simulink model "MLP_Final_Golden"  (R2015b)
settings: Solver=FixedStepDiscrete  SolverMode=SingleTasking  StartTime=0.0  StopTime=1e-2  RelTol=1e-3
undefined symbols (not defined in the file): input_sample_time, system_sample_time
libraries: shlslibv1 x1948
(part 5 of 11)

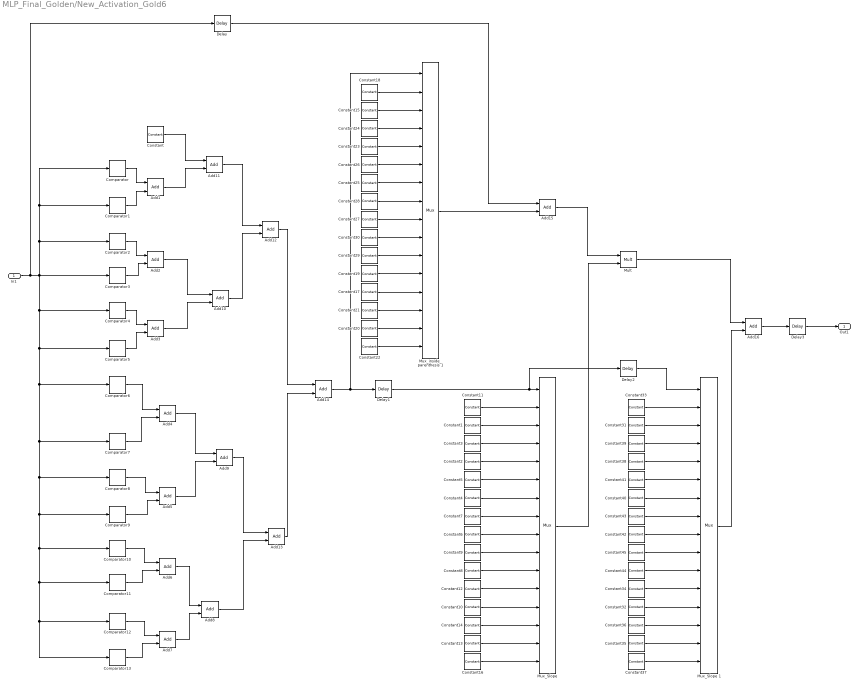
== system MLP_Final_Golden/New_Activation_Gold6 ==
  In1 : Inport
  Add{1..14} (14 alike) : shlslibv1/Math Functions/Add  syn_add_opr=++  syn_out_f=Specify  syn_out_wl=5  syn_out_fl=0  syn_out_dt=unsigned  syn_out_sat=off  syn_out_rnd=Nearest  synBlockType=primitive  synLatency=0  synBlockId=96  syn_sum_of_rows=off  syn_inh_port=off  syn_inh_st=on  syn_inh_stf=1  syn_en_pipe=on  syn_pipe_stg=3  syn_flow_ctrl=off
  Add15 : shlslibv1/Math Functions/Add  syn_add_opr=+-  syn_out_f=Specify  syn_out_wl=32  syn_out_fl=16  syn_out_dt=signed  syn_out_sat=off  syn_out_rnd=Floor (Truncate)  synBlockType=primitive  synLatency=0  synBlockId=96  syn_sum_of_rows=off  syn_inh_port=off  syn_inh_st=on  syn_inh_stf=1  syn_en_pipe=on  syn_pipe_stg=3  syn_flow_ctrl=off
  Add16 : shlslibv1/Math Functions/Add  syn_add_opr=++  syn_out_f=Specify  syn_out_wl=32  syn_out_fl=16  syn_out_dt=signed  syn_out_sat=off  syn_out_rnd=Floor (Truncate)  synBlockType=primitive  synLatency=0  synBlockId=96  syn_sum_of_rows=off  syn_inh_port=off  syn_inh_st=on  syn_inh_stf=1  syn_en_pipe=on  syn_pipe_stg=3  syn_flow_ctrl=off
  Comparator : shlslibv1/Math Functions/Comparator  syn_comp_opr=a>=b  syn_comp_const=on  syn_comp_val=6.5  syn_en_se=off  synBlockType=primitive  synLatency=0  synBlockId=14
  Comparator1 : shlslibv1/Math Functions/Comparator  syn_comp_opr=a>=b  syn_comp_const=on  syn_comp_val=5.5  syn_en_se=off  synBlockType=primitive  synLatency=0  synBlockId=14
  Comparator10 : shlslibv1/Math Functions/Comparator  syn_comp_opr=a>=b  syn_comp_const=on  syn_comp_val=-3.5  syn_en_se=off  synBlockType=primitive  synLatency=0  synBlockId=14
  Comparator11 : shlslibv1/Math Functions/Comparator  syn_comp_opr=a>=b  syn_comp_const=on  syn_comp_val=-4.5  syn_en_se=off  synBlockType=primitive  synLatency=0  synBlockId=14
  Comparator12 : shlslibv1/Math Functions/Comparator  syn_comp_opr=a>=b  syn_comp_const=on  syn_comp_val=-5.5  syn_en_se=off  synBlockType=primitive  synLatency=0  synBlockId=14
  Comparator13 : shlslibv1/Math Functions/Comparator  syn_comp_opr=a>=b  syn_comp_const=on  syn_comp_val=-6.5  syn_en_se=off  synBlockType=primitive  synLatency=0  synBlockId=14
  Comparator2 : shlslibv1/Math Functions/Comparator  syn_comp_opr=a>=b  syn_comp_const=on  syn_comp_val=4.5  syn_en_se=off  synBlockType=primitive  synLatency=0  synBlockId=14
  Comparator3 : shlslibv1/Math Functions/Comparator  syn_comp_opr=a>=b  syn_comp_const=on  syn_comp_val=3.5  syn_en_se=off  synBlockType=primitive  synLatency=0  synBlockId=14
  Comparator4 : shlslibv1/Math Functions/Comparator  syn_comp_opr=a>=b  syn_comp_const=on  syn_comp_val=2.5  syn_en_se=off  synBlockType=primitive  synLatency=0  synBlockId=14
  Comparator5 : shlslibv1/Math Functions/Comparator  syn_comp_opr=a>=b  syn_comp_const=on  syn_comp_val=1.5  syn_en_se=off  synBlockType=primitive  synLatency=0  synBlockId=14
  Comparator6 : shlslibv1/Math Functions/Comparator  syn_comp_opr=a>=b  syn_comp_const=on  syn_comp_val=0.5  syn_en_se=off  synBlockType=primitive  synLatency=0  synBlockId=14
  Comparator7 : shlslibv1/Math Functions/Comparator  syn_comp_opr=a>=b  syn_comp_const=on  syn_comp_val=-0.5  syn_en_se=off  synBlockType=primitive  synLatency=0  synBlockId=14
  Comparator8 : shlslibv1/Math Functions/Comparator  syn_comp_opr=a>=b  syn_comp_const=on  syn_comp_val=-1.5  syn_en_se=off  synBlockType=primitive  synLatency=0  synBlockId=14
  Comparator9 : shlslibv1/Math Functions/Comparator  syn_comp_opr=a>=b  syn_comp_const=on  syn_comp_val=-2.5  syn_en_se=off  synBlockType=primitive  synLatency=0  synBlockId=14
  Constant : shlslibv1/Sources/Constant  syn_cst_val=0  syn_cst_format=Specify  syn_cst_wl=5  syn_cst_fl=0  syn_cst_dt=unsigned  syn_cst_rnd=on  syn_cst_st=-1  synBlockType=primitive  synLatency=0  synBlockId=15
  Constant1 : shlslibv1/Sources/Constant  syn_cst_val=0.0025  syn_cst_format=Specify  syn_cst_wl=32  syn_cst_fl=16  syn_cst_dt=unsigned  syn_cst_rnd=on  syn_cst_st=-1  synBlockType=primitive  synLatency=0  synBlockId=15
  Constant10 : shlslibv1/Sources/Constant  syn_cst_val=0.0177  syn_cst_format=Specify  syn_cst_wl=32  syn_cst_fl=16  syn_cst_dt=unsigned  syn_cst_rnd=on  syn_cst_st=-1  synBlockType=primitive  synLatency=0  synBlockId=15
  Constant{11,16,18,22,33} (5 alike) : shlslibv1/Sources/Constant  syn_cst_val=0  syn_cst_format=Specify  syn_cst_wl=32  syn_cst_fl=16  syn_cst_dt=unsigned  syn_cst_rnd=on  syn_cst_st=-1  synBlockType=primitive  synLatency=0  synBlockId=15
  Constant12 : shlslibv1/Sources/Constant  syn_cst_val=0.0452  syn_cst_format=Specify  syn_cst_wl=32  syn_cst_fl=16  syn_cst_dt=unsigned  syn_cst_rnd=on  syn_cst_st=-1  synBlockType=primitive  synLatency=0  synBlockId=15
  Constant13 : shlslibv1/Sources/Constant  syn_cst_val=0.0025  syn_cst_format=Specify  syn_cst_wl=32  syn_cst_fl=16  syn_cst_dt=unsigned  syn_cst_rnd=on  syn_cst_st=-1  synBlockType=primitive  synLatency=0  synBlockId=15
  Constant14 : shlslibv1/Sources/Constant  syn_cst_val=0.0066  syn_cst_format=Specify  syn_cst_wl=32  syn_cst_fl=16  syn_cst_dt=unsigned  syn_cst_rnd=on  syn_cst_st=-1  synBlockType=primitive  synLatency=0  synBlockId=15
  Constant15 : shlslibv1/Sources/Constant  syn_cst_val=-6.5  syn_cst_format=Specify  syn_cst_wl=32  syn_cst_fl=16  syn_cst_dt=unsigned  syn_cst_rnd=on  syn_cst_st=-1  synBlockType=primitive  synLatency=0  synBlockId=15
  Constant17 : shlslibv1/Sources/Constant  syn_cst_val=3.5  syn_cst_format=Specify  syn_cst_wl=32  syn_cst_fl=16  syn_cst_dt=unsigned  syn_cst_rnd=on  syn_cst_st=-1  synBlockType=primitive  synLatency=0  synBlockId=15
  Constant19 : shlslibv1/Sources/Constant  syn_cst_val=2.5  syn_cst_format=Specify  syn_cst_wl=32  syn_cst_fl=16  syn_cst_dt=unsigned  syn_cst_rnd=on  syn_cst_st=-1  synBlockType=primitive  synLatency=0  synBlockId=15
  Constant2 : shlslibv1/Sources/Constant  syn_cst_val=0.0177  syn_cst_format=Specify  syn_cst_wl=32  syn_cst_fl=16  syn_cst_dt=unsigned  syn_cst_rnd=on  syn_cst_st=-1  synBlockType=primitive  synLatency=0  synBlockId=15
  Constant20 : shlslibv1/Sources/Constant  syn_cst_val=5.5  syn_cst_format=Specify  syn_cst_wl=32  syn_cst_fl=16  syn_cst_dt=unsigned  syn_cst_rnd=on  syn_cst_st=-1  synBlockType=primitive  synLatency=0  synBlockId=15
  Constant21 : shlslibv1/Sources/Constant  syn_cst_val=4.5  syn_cst_format=Specify  syn_cst_wl=32  syn_cst_fl=16  syn_cst_dt=unsigned  syn_cst_rnd=on  syn_cst_st=-1  synBlockType=primitive  synLatency=0  synBlockId=15
  Constant23 : shlslibv1/Sources/Constant  syn_cst_val=-4.5  syn_cst_format=Specify  syn_cst_wl=32  syn_cst_fl=16  syn_cst_dt=unsigned  syn_cst_rnd=on  syn_cst_st=-1  synBlockType=primitive  synLatency=0  synBlockId=15
  Constant24 : shlslibv1/Sources/Constant  syn_cst_val=-5.5  syn_cst_format=Specify  syn_cst_wl=32  syn_cst_fl=16  syn_cst_dt=unsigned  syn_cst_rnd=on  syn_cst_st=-1  synBlockType=primitive  synLatency=0  synBlockId=15
  Constant25 : shlslibv1/Sources/Constant  syn_cst_val=-2.5  syn_cst_format=Specify  syn_cst_wl=32  syn_cst_fl=16  syn_cst_dt=unsigned  syn_cst_rnd=on  syn_cst_st=-1  synBlockType=primitive  synLatency=0  synBlockId=15
  Constant26 : shlslibv1/Sources/Constant  syn_cst_val=-3.5  syn_cst_format=Specify  syn_cst_wl=32  syn_cst_fl=16  syn_cst_dt=unsigned  syn_cst_rnd=on  syn_cst_st=-1  synBlockType=primitive  synLatency=0  synBlockId=15
  Constant27 : shlslibv1/Sources/Constant  syn_cst_val=-0.5  syn_cst_format=Specify  syn_cst_wl=32  syn_cst_fl=16  syn_cst_dt=unsigned  syn_cst_rnd=on  syn_cst_st=-1  synBlockType=primitive  synLatency=0  synBlockId=15
  Constant28 : shlslibv1/Sources/Constant  syn_cst_val=-1.5  syn_cst_format=Specify  syn_cst_wl=32  syn_cst_fl=16  syn_cst_dt=unsigned  syn_cst_rnd=on  syn_cst_st=-1  synBlockType=primitive  synLatency=0  synBlockId=15
  Constant29 : shlslibv1/Sources/Constant  syn_cst_val=1.5  syn_cst_format=Specify  syn_cst_wl=32  syn_cst_fl=16  syn_cst_dt=unsigned  syn_cst_rnd=on  syn_cst_st=-1  synBlockType=primitive  synLatency=0  synBlockId=15
  Constant3 : shlslibv1/Sources/Constant  syn_cst_val=0.0066  syn_cst_format=Specify  syn_cst_wl=32  syn_cst_fl=16  syn_cst_dt=unsigned  syn_cst_rnd=on  syn_cst_st=-1  synBlockType=primitive  synLatency=0  synBlockId=15
  Constant30 : shlslibv1/Sources/Constant  syn_cst_val=0.5  syn_cst_format=Specify  syn_cst_wl=32  syn_cst_fl=16  syn_cst_dt=unsigned  syn_cst_rnd=on  syn_cst_st=-1  synBlockType=primitive  synLatency=0  synBlockId=15
  Constant31 : shlslibv1/Sources/Constant  syn_cst_val=0.0015  syn_cst_format=Specify  syn_cst_wl=32  syn_cst_fl=16  syn_cst_dt=unsigned  syn_cst_rnd=on  syn_cst_st=-1  synBlockType=primitive  synLatency=0  synBlockId=15
  Constant32 : shlslibv1/Sources/Constant  syn_cst_val=0.9707  syn_cst_format=Specify  syn_cst_wl=32  syn_cst_fl=16  syn_cst_dt=unsigned  syn_cst_rnd=on  syn_cst_st=-1  synBlockType=primitive  synLatency=0  synBlockId=15
  Constant34 : shlslibv1/Sources/Constant  syn_cst_val=0.9241  syn_cst_format=Specify  syn_cst_wl=32  syn_cst_fl=16  syn_cst_dt=unsigned  syn_cst_rnd=on  syn_cst_st=-1  synBlockType=primitive  synLatency=0  synBlockId=15
  Constant35 : shlslibv1/Sources/Constant  syn_cst_val=0.9959  syn_cst_format=Specify  syn_cst_wl=32  syn_cst_fl=16  syn_cst_dt=unsigned  syn_cst_rnd=on  syn_cst_st=-1  synBlockType=primitive  synLatency=0  synBlockId=15
  Constant36 : shlslibv1/Sources/Constant  syn_cst_val=0.9890  syn_cst_format=Specify  syn_cst_wl=32  syn_cst_fl=16  syn_cst_dt=unsigned  syn_cst_rnd=on  syn_cst_st=-1  synBlockType=primitive  synLatency=0  synBlockId=15
  Constant37 : shlslibv1/Sources/Constant  syn_cst_val=1  syn_cst_format=Specify  syn_cst_wl=32  syn_cst_fl=16  syn_cst_dt=unsigned  syn_cst_rnd=on  syn_cst_st=-1  synBlockType=primitive  synLatency=0  synBlockId=15
  Constant38 : shlslibv1/Sources/Constant  syn_cst_val=0.011  syn_cst_format=Specify  syn_cst_wl=32  syn_cst_fl=16  syn_cst_dt=unsigned  syn_cst_rnd=on  syn_cst_st=-1  synBlockType=primitive  synLatency=0  synBlockId=15
  Constant39 : shlslibv1/Sources/Constant  syn_cst_val=0.0041  syn_cst_format=Specify  syn_cst_wl=32  syn_cst_fl=16  syn_cst_dt=unsigned  syn_cst_rnd=on  syn_cst_st=-1  synBlockType=primitive  synLatency=0  synBlockId=15
  Constant4 : shlslibv1/Sources/Constant  syn_cst_val=0.1050  syn_cst_format=Specify  syn_cst_wl=32  syn_cst_fl=16  syn_cst_dt=unsigned  syn_cst_rnd=on  syn_cst_st=-1  synBlockType=primitive  synLatency=0  synBlockId=15
  Constant40 : shlslibv1/Sources/Constant  syn_cst_val=0.0759  syn_cst_format=Specify  syn_cst_wl=32  syn_cst_fl=16  syn_cst_dt=unsigned  syn_cst_rnd=on  syn_cst_st=-1  synBlockType=primitive  synLatency=0  synBlockId=15
  Constant41 : shlslibv1/Sources/Constant  syn_cst_val=0.0293  syn_cst_format=Specify  syn_cst_wl=32  syn_cst_fl=16  syn_cst_dt=unsigned  syn_cst_rnd=on  syn_cst_st=-1  synBlockType=primitive  synLatency=0  synBlockId=15
  Constant42 : shlslibv1/Sources/Constant  syn_cst_val=0.3775  syn_cst_format=Specify  syn_cst_wl=32  syn_cst_fl=16  syn_cst_dt=unsigned  syn_cst_rnd=on  syn_cst_st=-1  synBlockType=primitive  synLatency=0  synBlockId=15
  Constant43 : shlslibv1/Sources/Constant  syn_cst_val=0.1824  syn_cst_format=Specify  syn_cst_wl=32  syn_cst_fl=16  syn_cst_dt=unsigned  syn_cst_rnd=on  syn_cst_st=-1  synBlockType=primitive  synLatency=0  synBlockId=15
  Constant44 : shlslibv1/Sources/Constant  syn_cst_val=0.8176  syn_cst_format=Specify  syn_cst_wl=32  syn_cst_fl=16  syn_cst_dt=unsigned  syn_cst_rnd=on  syn_cst_st=-1  synBlockType=primitive  synLatency=0  synBlockId=15
  Constant45 : shlslibv1/Sources/Constant  syn_cst_val=0.6225  syn_cst_format=Specify  syn_cst_wl=32  syn_cst_fl=16  syn_cst_dt=unsigned  syn_cst_rnd=on  syn_cst_st=-1  synBlockType=primitive  synLatency=0  synBlockId=15
  Constant5 : shlslibv1/Sources/Constant  syn_cst_val=0.0452  syn_cst_format=Specify  syn_cst_wl=32  syn_cst_fl=16  syn_cst_dt=unsigned  syn_cst_rnd=on  syn_cst_st=-1  synBlockType=primitive  synLatency=0  synBlockId=15
  Constant6 : shlslibv1/Sources/Constant  syn_cst_val=0.25  syn_cst_format=Specify  syn_cst_wl=32  syn_cst_fl=16  syn_cst_dt=unsigned  syn_cst_rnd=on  syn_cst_st=-1  synBlockType=primitive  synLatency=0  synBlockId=15
  Constant7 : shlslibv1/Sources/Constant  syn_cst_val=0.1966  syn_cst_format=Specify  syn_cst_wl=32  syn_cst_fl=16  syn_cst_dt=unsigned  syn_cst_rnd=on  syn_cst_st=-1  synBlockType=primitive  synLatency=0  synBlockId=15
  Constant8 : shlslibv1/Sources/Constant  syn_cst_val=0.1050  syn_cst_format=Specify  syn_cst_wl=32  syn_cst_fl=16  syn_cst_dt=unsigned  syn_cst_rnd=on  syn_cst_st=-1  synBlockType=primitive  synLatency=0  synBlockId=15
  Constant9 : shlslibv1/Sources/Constant  syn_cst_val=0.1966  syn_cst_format=Specify  syn_cst_wl=32  syn_cst_fl=16  syn_cst_dt=unsigned  syn_cst_rnd=on  syn_cst_st=-1  synBlockType=primitive  synLatency=0  synBlockId=15
  Delay : shlslibv1/Memories/Delay  syn_delay_val=12  synBlockType=primitive  synLatency=12  synBlockId=104
  Delay1 : shlslibv1/Memories/Delay  syn_delay_val=3  synBlockType=primitive  synLatency=3  synBlockId=104
  Delay2 : shlslibv1/Memories/Delay  syn_delay_val=6  synBlockType=primitive  synLatency=6  synBlockId=104
  Delay3 : shlslibv1/Memories/Delay  syn_delay_val=5  synBlockType=primitive  synLatency=5  synBlockId=104
  Mult : shlslibv1/Math Functions/Mult  syn_out_f=Specify  syn_out_wl=32  syn_out_fl=16  syn_out_dt=signed  syn_out_sat=off  syn_out_rnd=Floor (Truncate)  syn_inh_port=off  syn_inh_st=off  syn_inh_stf=1  syn_en_pipe=on  syn_pipe_stg=6  syn_flow_ctrl=off  synBlockType=primitive  synLatency=0  synBlockId=3  syn_opr_mode=1
  "Mux_Slope " : shlslibv1/Signal Operations/Mux  syn_in_nb=15  syn_out_f=Specify  syn_out_wl=32  syn_out_fl=16  syn_out_dt=signed  syn_en_se=off  synBlockType=primitive  synLatency=0  synBlockId=16
  Mux_Slope 1 : shlslibv1/Signal Operations/Mux  syn_in_nb=15  syn_out_f=Specify  syn_out_wl=32  syn_out_fl=16  syn_out_dt=signed  syn_en_se=off  synBlockType=primitive  synLatency=0  synBlockId=16
  Mux_inside_parenthesis 1 : shlslibv1/Signal Operations/Mux  syn_in_nb=15  syn_out_f=Specify  syn_out_wl=32  syn_out_fl=16  syn_out_dt=signed  syn_en_se=off  synBlockType=primitive  synLatency=0  synBlockId=16
  Out1 : Outport
  wires:
  Add12/1 -> Add14/1
  Constant14/1 -> "Mux_Slope "/14
  Constant13/1 -> "Mux_Slope "/15
  Comparator/1 -> Add1/1
  Add4/1 -> Add9/1
  Delay/1 -> Add15/1
  Constant5/1 -> "Mux_Slope "/6
  Comparator13/1 -> Add7/2
  Constant/1 -> Add11/1
  Constant29/1 -> Mux_inside_parenthesis 1/11
  Add2/1 -> Add10/1
  Add13/1 -> Add14/2
  Constant20/1 -> Mux_inside_parenthesis 1/15
  Constant23/1 -> Mux_inside_parenthesis 1/5
  Constant17/1 -> Mux_inside_parenthesis 1/13
  Add6/1 -> Add8/1
  Comparator9/1 -> Add5/2
  Constant3/1 -> "Mux_Slope "/4
  Constant2/1 -> "Mux_Slope "/5
  In1/1 -> Delay/1, Comparator7/1, Comparator8/1, Comparator12/1, Comparator13/1, Comparator11/1, Comparator10/1, Comparator9/1, Comparator6/1, Comparator5/1, Comparator4/1, Comparator3/1, Comparator2/1, Comparator1/1, Comparator/1
  Comparator2/1 -> Add2/1
  Comparator11/1 -> Add6/2
  Add11/1 -> Add12/1
  Comparator1/1 -> Add1/2
  Constant22/1 -> Mux_inside_parenthesis 1/16
  Add3/1 -> Add10/2
  Add10/1 -> Add12/2
  Comparator12/1 -> Add7/1
  Comparator8/1 -> Add5/1
  Constant9/1 -> "Mux_Slope "/10
  Add7/1 -> Add8/2
  Add14/1 -> Delay1/1, Mux_inside_parenthesis 1/1
  Constant42/1 -> Mux_Slope 1/9
  Constant1/1 -> "Mux_Slope "/3
  Constant16/1 -> "Mux_Slope "/16
  Constant24/1 -> Mux_inside_parenthesis 1/4
  Constant19/1 -> Mux_inside_parenthesis 1/12
  Constant39/1 -> Mux_Slope 1/4
  Constant41/1 -> Mux_Slope 1/6
  Constant38/1 -> Mux_Slope 1/5
  Delay1/1 -> Delay2/1, "Mux_Slope "/1
  Constant30/1 -> Mux_inside_parenthesis 1/10
  Constant45/1 -> Mux_Slope 1/10
  Constant44/1 -> Mux_Slope 1/11
  Constant34/1 -> Mux_Slope 1/12
  Constant28/1 -> Mux_inside_parenthesis 1/8
  Constant26/1 -> Mux_inside_parenthesis 1/6
  Constant21/1 -> Mux_inside_parenthesis 1/14
  Constant8/1 -> "Mux_Slope "/11
  Constant12/1 -> "Mux_Slope "/12
  Constant10/1 -> "Mux_Slope "/13
  Comparator5/1 -> Add3/2
  Constant27/1 -> Mux_inside_parenthesis 1/9
  Constant18/1 -> Mux_inside_parenthesis 1/2
  Comparator4/1 -> Add3/1
  Comparator10/1 -> Add6/1
  Constant11/1 -> "Mux_Slope "/2
  "Mux_Slope "/1 -> Mult/2
  Constant15/1 -> Mux_inside_parenthesis 1/3
  Constant32/1 -> Mux_Slope 1/13
  Constant36/1 -> Mux_Slope 1/14
  Constant35/1 -> Mux_Slope 1/15
  Constant31/1 -> Mux_Slope 1/3
  Constant25/1 -> Mux_inside_parenthesis 1/7
  Constant37/1 -> Mux_Slope 1/16
  Constant33/1 -> Mux_Slope 1/2
  Constant43/1 -> Mux_Slope 1/8
  Constant40/1 -> Mux_Slope 1/7
  Delay2/1 -> Mux_Slope 1/1
  Mult/1 -> Add16/1
  Add1/1 -> Add11/2
  Add9/1 -> Add13/1
  Constant6/1 -> "Mux_Slope "/9
  Constant4/1 -> "Mux_Slope "/7
  Add5/1 -> Add9/2
  Comparator6/1 -> Add4/1
  Comparator7/1 -> Add4/2
  Comparator3/1 -> Add2/2
  Mux_Slope 1/1 -> Add16/2
  Add8/1 -> Add13/2
  Mux_inside_parenthesis 1/1 -> Add15/2
  Constant7/1 -> "Mux_Slope "/8
  Add15/1 -> Mult/1
  Delay3/1 -> Out1/1
  Add16/1 -> Delay3/1

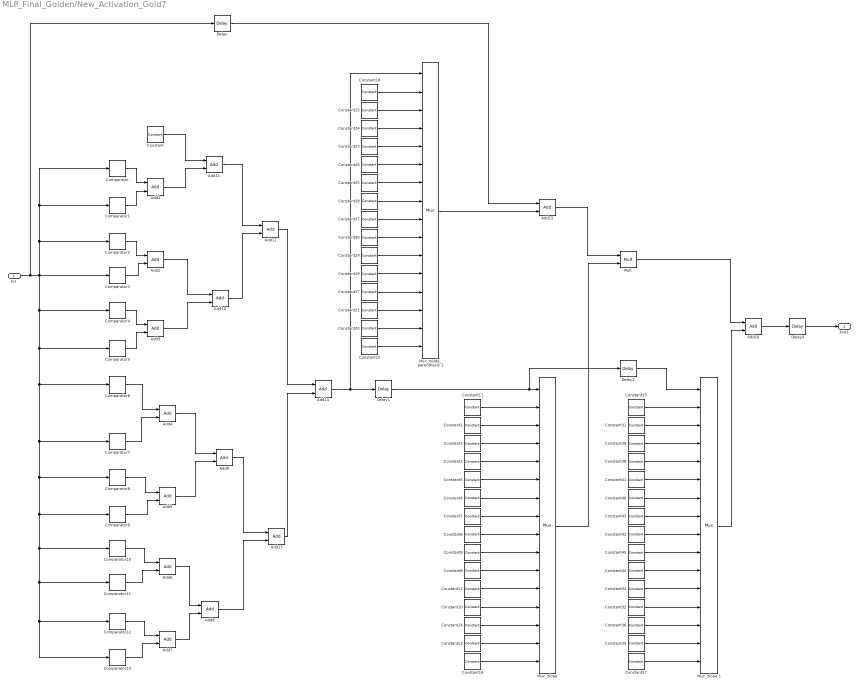
== system MLP_Final_Golden/New_Activation_Gold7 ==
  In1 : Inport
  Add{1..14} (14 alike) : shlslibv1/Math Functions/Add  syn_add_opr=++  syn_out_f=Specify  syn_out_wl=5  syn_out_fl=0  syn_out_dt=unsigned  syn_out_sat=off  syn_out_rnd=Nearest  synBlockType=primitive  synLatency=0  synBlockId=96  syn_sum_of_rows=off  syn_inh_port=off  syn_inh_st=on  syn_inh_stf=1  syn_en_pipe=on  syn_pipe_stg=3  syn_flow_ctrl=off
  Add15 : shlslibv1/Math Functions/Add  syn_add_opr=+-  syn_out_f=Specify  syn_out_wl=32  syn_out_fl=16  syn_out_dt=signed  syn_out_sat=off  syn_out_rnd=Floor (Truncate)  synBlockType=primitive  synLatency=0  synBlockId=96  syn_sum_of_rows=off  syn_inh_port=off  syn_inh_st=on  syn_inh_stf=1  syn_en_pipe=on  syn_pipe_stg=3  syn_flow_ctrl=off
  Add16 : shlslibv1/Math Functions/Add  syn_add_opr=++  syn_out_f=Specify  syn_out_wl=32  syn_out_fl=16  syn_out_dt=signed  syn_out_sat=off  syn_out_rnd=Floor (Truncate)  synBlockType=primitive  synLatency=0  synBlockId=96  syn_sum_of_rows=off  syn_inh_port=off  syn_inh_st=on  syn_inh_stf=1  syn_en_pipe=on  syn_pipe_stg=3  syn_flow_ctrl=off
  Comparator : shlslibv1/Math Functions/Comparator  syn_comp_opr=a>=b  syn_comp_const=on  syn_comp_val=6.5  syn_en_se=off  synBlockType=primitive  synLatency=0  synBlockId=14
  Comparator1 : shlslibv1/Math Functions/Comparator  syn_comp_opr=a>=b  syn_comp_const=on  syn_comp_val=5.5  syn_en_se=off  synBlockType=primitive  synLatency=0  synBlockId=14
  Comparator10 : shlslibv1/Math Functions/Comparator  syn_comp_opr=a>=b  syn_comp_const=on  syn_comp_val=-3.5  syn_en_se=off  synBlockType=primitive  synLatency=0  synBlockId=14
  Comparator11 : shlslibv1/Math Functions/Comparator  syn_comp_opr=a>=b  syn_comp_const=on  syn_comp_val=-4.5  syn_en_se=off  synBlockType=primitive  synLatency=0  synBlockId=14
  Comparator12 : shlslibv1/Math Functions/Comparator  syn_comp_opr=a>=b  syn_comp_const=on  syn_comp_val=-5.5  syn_en_se=off  synBlockType=primitive  synLatency=0  synBlockId=14
  Comparator13 : shlslibv1/Math Functions/Comparator  syn_comp_opr=a>=b  syn_comp_const=on  syn_comp_val=-6.5  syn_en_se=off  synBlockType=primitive  synLatency=0  synBlockId=14
  Comparator2 : shlslibv1/Math Functions/Comparator  syn_comp_opr=a>=b  syn_comp_const=on  syn_comp_val=4.5  syn_en_se=off  synBlockType=primitive  synLatency=0  synBlockId=14
  Comparator3 : shlslibv1/Math Functions/Comparator  syn_comp_opr=a>=b  syn_comp_const=on  syn_comp_val=3.5  syn_en_se=off  synBlockType=primitive  synLatency=0  synBlockId=14
  Comparator4 : shlslibv1/Math Functions/Comparator  syn_comp_opr=a>=b  syn_comp_const=on  syn_comp_val=2.5  syn_en_se=off  synBlockType=primitive  synLatency=0  synBlockId=14
  Comparator5 : shlslibv1/Math Functions/Comparator  syn_comp_opr=a>=b  syn_comp_const=on  syn_comp_val=1.5  syn_en_se=off  synBlockType=primitive  synLatency=0  synBlockId=14
  Comparator6 : shlslibv1/Math Functions/Comparator  syn_comp_opr=a>=b  syn_comp_const=on  syn_comp_val=0.5  syn_en_se=off  synBlockType=primitive  synLatency=0  synBlockId=14
  Comparator7 : shlslibv1/Math Functions/Comparator  syn_comp_opr=a>=b  syn_comp_const=on  syn_comp_val=-0.5  syn_en_se=off  synBlockType=primitive  synLatency=0  synBlockId=14
  Comparator8 : shlslibv1/Math Functions/Comparator  syn_comp_opr=a>=b  syn_comp_const=on  syn_comp_val=-1.5  syn_en_se=off  synBlockType=primitive  synLatency=0  synBlockId=14
  Comparator9 : shlslibv1/Math Functions/Comparator  syn_comp_opr=a>=b  syn_comp_const=on  syn_comp_val=-2.5  syn_en_se=off  synBlockType=primitive  synLatency=0  synBlockId=14
  Constant : shlslibv1/Sources/Constant  syn_cst_val=0  syn_cst_format=Specify  syn_cst_wl=5  syn_cst_fl=0  syn_cst_dt=unsigned  syn_cst_rnd=on  syn_cst_st=-1  synBlockType=primitive  synLatency=0  synBlockId=15
  Constant1 : shlslibv1/Sources/Constant  syn_cst_val=0.0025  syn_cst_format=Specify  syn_cst_wl=32  syn_cst_fl=16  syn_cst_dt=unsigned  syn_cst_rnd=on  syn_cst_st=-1  synBlockType=primitive  synLatency=0  synBlockId=15
  Constant10 : shlslibv1/Sources/Constant  syn_cst_val=0.0177  syn_cst_format=Specify  syn_cst_wl=32  syn_cst_fl=16  syn_cst_dt=unsigned  syn_cst_rnd=on  syn_cst_st=-1  synBlockType=primitive  synLatency=0  synBlockId=15
  Constant{11,16,18,22,33} (5 alike) : shlslibv1/Sources/Constant  syn_cst_val=0  syn_cst_format=Specify  syn_cst_wl=32  syn_cst_fl=16  syn_cst_dt=unsigned  syn_cst_rnd=on  syn_cst_st=-1  synBlockType=primitive  synLatency=0  synBlockId=15
  Constant12 : shlslibv1/Sources/Constant  syn_cst_val=0.0452  syn_cst_format=Specify  syn_cst_wl=32  syn_cst_fl=16  syn_cst_dt=unsigned  syn_cst_rnd=on  syn_cst_st=-1  synBlockType=primitive  synLatency=0  synBlockId=15
  Constant13 : shlslibv1/Sources/Constant  syn_cst_val=0.0025  syn_cst_format=Specify  syn_cst_wl=32  syn_cst_fl=16  syn_cst_dt=unsigned  syn_cst_rnd=on  syn_cst_st=-1  synBlockType=primitive  synLatency=0  synBlockId=15
  Constant14 : shlslibv1/Sources/Constant  syn_cst_val=0.0066  syn_cst_format=Specify  syn_cst_wl=32  syn_cst_fl=16  syn_cst_dt=unsigned  syn_cst_rnd=on  syn_cst_st=-1  synBlockType=primitive  synLatency=0  synBlockId=15
  Constant15 : shlslibv1/Sources/Constant  syn_cst_val=-6.5  syn_cst_format=Specify  syn_cst_wl=32  syn_cst_fl=16  syn_cst_dt=unsigned  syn_cst_rnd=on  syn_cst_st=-1  synBlockType=primitive  synLatency=0  synBlockId=15
  Constant17 : shlslibv1/Sources/Constant  syn_cst_val=3.5  syn_cst_format=Specify  syn_cst_wl=32  syn_cst_fl=16  syn_cst_dt=unsigned  syn_cst_rnd=on  syn_cst_st=-1  synBlockType=primitive  synLatency=0  synBlockId=15
  Constant19 : shlslibv1/Sources/Constant  syn_cst_val=2.5  syn_cst_format=Specify  syn_cst_wl=32  syn_cst_fl=16  syn_cst_dt=unsigned  syn_cst_rnd=on  syn_cst_st=-1  synBlockType=primitive  synLatency=0  synBlockId=15
  Constant2 : shlslibv1/Sources/Constant  syn_cst_val=0.0177  syn_cst_format=Specify  syn_cst_wl=32  syn_cst_fl=16  syn_cst_dt=unsigned  syn_cst_rnd=on  syn_cst_st=-1  synBlockType=primitive  synLatency=0  synBlockId=15
  Constant20 : shlslibv1/Sources/Constant  syn_cst_val=5.5  syn_cst_format=Specify  syn_cst_wl=32  syn_cst_fl=16  syn_cst_dt=unsigned  syn_cst_rnd=on  syn_cst_st=-1  synBlockType=primitive  synLatency=0  synBlockId=15
  Constant21 : shlslibv1/Sources/Constant  syn_cst_val=4.5  syn_cst_format=Specify  syn_cst_wl=32  syn_cst_fl=16  syn_cst_dt=unsigned  syn_cst_rnd=on  syn_cst_st=-1  synBlockType=primitive  synLatency=0  synBlockId=15
  Constant23 : shlslibv1/Sources/Constant  syn_cst_val=-4.5  syn_cst_format=Specify  syn_cst_wl=32  syn_cst_fl=16  syn_cst_dt=unsigned  syn_cst_rnd=on  syn_cst_st=-1  synBlockType=primitive  synLatency=0  synBlockId=15
  Constant24 : shlslibv1/Sources/Constant  syn_cst_val=-5.5  syn_cst_format=Specify  syn_cst_wl=32  syn_cst_fl=16  syn_cst_dt=unsigned  syn_cst_rnd=on  syn_cst_st=-1  synBlockType=primitive  synLatency=0  synBlockId=15
  Constant25 : shlslibv1/Sources/Constant  syn_cst_val=-2.5  syn_cst_format=Specify  syn_cst_wl=32  syn_cst_fl=16  syn_cst_dt=unsigned  syn_cst_rnd=on  syn_cst_st=-1  synBlockType=primitive  synLatency=0  synBlockId=15
  Constant26 : shlslibv1/Sources/Constant  syn_cst_val=-3.5  syn_cst_format=Specify  syn_cst_wl=32  syn_cst_fl=16  syn_cst_dt=unsigned  syn_cst_rnd=on  syn_cst_st=-1  synBlockType=primitive  synLatency=0  synBlockId=15
  Constant27 : shlslibv1/Sources/Constant  syn_cst_val=-0.5  syn_cst_format=Specify  syn_cst_wl=32  syn_cst_fl=16  syn_cst_dt=unsigned  syn_cst_rnd=on  syn_cst_st=-1  synBlockType=primitive  synLatency=0  synBlockId=15
  Constant28 : shlslibv1/Sources/Constant  syn_cst_val=-1.5  syn_cst_format=Specify  syn_cst_wl=32  syn_cst_fl=16  syn_cst_dt=unsigned  syn_cst_rnd=on  syn_cst_st=-1  synBlockType=primitive  synLatency=0  synBlockId=15
  Constant29 : shlslibv1/Sources/Constant  syn_cst_val=1.5  syn_cst_format=Specify  syn_cst_wl=32  syn_cst_fl=16  syn_cst_dt=unsigned  syn_cst_rnd=on  syn_cst_st=-1  synBlockType=primitive  synLatency=0  synBlockId=15
  Constant3 : shlslibv1/Sources/Constant  syn_cst_val=0.0066  syn_cst_format=Specify  syn_cst_wl=32  syn_cst_fl=16  syn_cst_dt=unsigned  syn_cst_rnd=on  syn_cst_st=-1  synBlockType=primitive  synLatency=0  synBlockId=15
  Constant30 : shlslibv1/Sources/Constant  syn_cst_val=0.5  syn_cst_format=Specify  syn_cst_wl=32  syn_cst_fl=16  syn_cst_dt=unsigned  syn_cst_rnd=on  syn_cst_st=-1  synBlockType=primitive  synLatency=0  synBlockId=15
  Constant31 : shlslibv1/Sources/Constant  syn_cst_val=0.0015  syn_cst_format=Specify  syn_cst_wl=32  syn_cst_fl=16  syn_cst_dt=unsigned  syn_cst_rnd=on  syn_cst_st=-1  synBlockType=primitive  synLatency=0  synBlockId=15
  Constant32 : shlslibv1/Sources/Constant  syn_cst_val=0.9707  syn_cst_format=Specify  syn_cst_wl=32  syn_cst_fl=16  syn_cst_dt=unsigned  syn_cst_rnd=on  syn_cst_st=-1  synBlockType=primitive  synLatency=0  synBlockId=15
  Constant34 : shlslibv1/Sources/Constant  syn_cst_val=0.9241  syn_cst_format=Specify  syn_cst_wl=32  syn_cst_fl=16  syn_cst_dt=unsigned  syn_cst_rnd=on  syn_cst_st=-1  synBlockType=primitive  synLatency=0  synBlockId=15
  Constant35 : shlslibv1/Sources/Constant  syn_cst_val=0.9959  syn_cst_format=Specify  syn_cst_wl=32  syn_cst_fl=16  syn_cst_dt=unsigned  syn_cst_rnd=on  syn_cst_st=-1  synBlockType=primitive  synLatency=0  synBlockId=15
  Constant36 : shlslibv1/Sources/Constant  syn_cst_val=0.9890  syn_cst_format=Specify  syn_cst_wl=32  syn_cst_fl=16  syn_cst_dt=unsigned  syn_cst_rnd=on  syn_cst_st=-1  synBlockType=primitive  synLatency=0  synBlockId=15
  Constant37 : shlslibv1/Sources/Constant  syn_cst_val=1  syn_cst_format=Specify  syn_cst_wl=32  syn_cst_fl=16  syn_cst_dt=unsigned  syn_cst_rnd=on  syn_cst_st=-1  synBlockType=primitive  synLatency=0  synBlockId=15
  Constant38 : shlslibv1/Sources/Constant  syn_cst_val=0.011  syn_cst_format=Specify  syn_cst_wl=32  syn_cst_fl=16  syn_cst_dt=unsigned  syn_cst_rnd=on  syn_cst_st=-1  synBlockType=primitive  synLatency=0  synBlockId=15
  Constant39 : shlslibv1/Sources/Constant  syn_cst_val=0.0041  syn_cst_format=Specify  syn_cst_wl=32  syn_cst_fl=16  syn_cst_dt=unsigned  syn_cst_rnd=on  syn_cst_st=-1  synBlockType=primitive  synLatency=0  synBlockId=15
  Constant4 : shlslibv1/Sources/Constant  syn_cst_val=0.1050  syn_cst_format=Specify  syn_cst_wl=32  syn_cst_fl=16  syn_cst_dt=unsigned  syn_cst_rnd=on  syn_cst_st=-1  synBlockType=primitive  synLatency=0  synBlockId=15
  Constant40 : shlslibv1/Sources/Constant  syn_cst_val=0.0759  syn_cst_format=Specify  syn_cst_wl=32  syn_cst_fl=16  syn_cst_dt=unsigned  syn_cst_rnd=on  syn_cst_st=-1  synBlockType=primitive  synLatency=0  synBlockId=15
  Constant41 : shlslibv1/Sources/Constant  syn_cst_val=0.0293  syn_cst_format=Specify  syn_cst_wl=32  syn_cst_fl=16  syn_cst_dt=unsigned  syn_cst_rnd=on  syn_cst_st=-1  synBlockType=primitive  synLatency=0  synBlockId=15
  Constant42 : shlslibv1/Sources/Constant  syn_cst_val=0.3775  syn_cst_format=Specify  syn_cst_wl=32  syn_cst_fl=16  syn_cst_dt=unsigned  syn_cst_rnd=on  syn_cst_st=-1  synBlockType=primitive  synLatency=0  synBlockId=15
  Constant43 : shlslibv1/Sources/Constant  syn_cst_val=0.1824  syn_cst_format=Specify  syn_cst_wl=32  syn_cst_fl=16  syn_cst_dt=unsigned  syn_cst_rnd=on  syn_cst_st=-1  synBlockType=primitive  synLatency=0  synBlockId=15
  Constant44 : shlslibv1/Sources/Constant  syn_cst_val=0.8176  syn_cst_format=Specify  syn_cst_wl=32  syn_cst_fl=16  syn_cst_dt=unsigned  syn_cst_rnd=on  syn_cst_st=-1  synBlockType=primitive  synLatency=0  synBlockId=15
  Constant45 : shlslibv1/Sources/Constant  syn_cst_val=0.6225  syn_cst_format=Specify  syn_cst_wl=32  syn_cst_fl=16  syn_cst_dt=unsigned  syn_cst_rnd=on  syn_cst_st=-1  synBlockType=primitive  synLatency=0  synBlockId=15
  Constant5 : shlslibv1/Sources/Constant  syn_cst_val=0.0452  syn_cst_format=Specify  syn_cst_wl=32  syn_cst_fl=16  syn_cst_dt=unsigned  syn_cst_rnd=on  syn_cst_st=-1  synBlockType=primitive  synLatency=0  synBlockId=15
  Constant6 : shlslibv1/Sources/Constant  syn_cst_val=0.25  syn_cst_format=Specify  syn_cst_wl=32  syn_cst_fl=16  syn_cst_dt=unsigned  syn_cst_rnd=on  syn_cst_st=-1  synBlockType=primitive  synLatency=0  synBlockId=15
  Constant7 : shlslibv1/Sources/Constant  syn_cst_val=0.1966  syn_cst_format=Specify  syn_cst_wl=32  syn_cst_fl=16  syn_cst_dt=unsigned  syn_cst_rnd=on  syn_cst_st=-1  synBlockType=primitive  synLatency=0  synBlockId=15
  Constant8 : shlslibv1/Sources/Constant  syn_cst_val=0.1050  syn_cst_format=Specify  syn_cst_wl=32  syn_cst_fl=16  syn_cst_dt=unsigned  syn_cst_rnd=on  syn_cst_st=-1  synBlockType=primitive  synLatency=0  synBlockId=15
  Constant9 : shlslibv1/Sources/Constant  syn_cst_val=0.1966  syn_cst_format=Specify  syn_cst_wl=32  syn_cst_fl=16  syn_cst_dt=unsigned  syn_cst_rnd=on  syn_cst_st=-1  synBlockType=primitive  synLatency=0  synBlockId=15
  Delay : shlslibv1/Memories/Delay  syn_delay_val=12  synBlockType=primitive  synLatency=12  synBlockId=104
  Delay1 : shlslibv1/Memories/Delay  syn_delay_val=3  synBlockType=primitive  synLatency=3  synBlockId=104
  Delay2 : shlslibv1/Memories/Delay  syn_delay_val=6  synBlockType=primitive  synLatency=6  synBlockId=104
  Delay3 : shlslibv1/Memories/Delay  syn_delay_val=5  synBlockType=primitive  synLatency=5  synBlockId=104
  Mult : shlslibv1/Math Functions/Mult  syn_out_f=Specify  syn_out_wl=32  syn_out_fl=16  syn_out_dt=signed  syn_out_sat=off  syn_out_rnd=Floor (Truncate)  syn_inh_port=off  syn_inh_st=off  syn_inh_stf=1  syn_en_pipe=on  syn_pipe_stg=6  syn_flow_ctrl=off  synBlockType=primitive  synLatency=0  synBlockId=3  syn_opr_mode=1
  "Mux_Slope " : shlslibv1/Signal Operations/Mux  syn_in_nb=15  syn_out_f=Specify  syn_out_wl=32  syn_out_fl=16  syn_out_dt=signed  syn_en_se=off  synBlockType=primitive  synLatency=0  synBlockId=16
  Mux_Slope 1 : shlslibv1/Signal Operations/Mux  syn_in_nb=15  syn_out_f=Specify  syn_out_wl=32  syn_out_fl=16  syn_out_dt=signed  syn_en_se=off  synBlockType=primitive  synLatency=0  synBlockId=16
  Mux_inside_parenthesis 1 : shlslibv1/Signal Operations/Mux  syn_in_nb=15  syn_out_f=Specify  syn_out_wl=32  syn_out_fl=16  syn_out_dt=signed  syn_en_se=off  synBlockType=primitive  synLatency=0  synBlockId=16
  Out1 : Outport
  wires:
  Add12/1 -> Add14/1
  Constant14/1 -> "Mux_Slope "/14
  Constant13/1 -> "Mux_Slope "/15
  Comparator/1 -> Add1/1
  Add4/1 -> Add9/1
  Delay/1 -> Add15/1
  Constant5/1 -> "Mux_Slope "/6
  Comparator13/1 -> Add7/2
  Constant/1 -> Add11/1
  Constant29/1 -> Mux_inside_parenthesis 1/11
  Add2/1 -> Add10/1
  Add13/1 -> Add14/2
  Constant20/1 -> Mux_inside_parenthesis 1/15
  Constant23/1 -> Mux_inside_parenthesis 1/5
  Constant17/1 -> Mux_inside_parenthesis 1/13
  Add6/1 -> Add8/1
  Comparator9/1 -> Add5/2
  Constant3/1 -> "Mux_Slope "/4
  Constant2/1 -> "Mux_Slope "/5
  In1/1 -> Delay/1, Comparator7/1, Comparator8/1, Comparator12/1, Comparator13/1, Comparator11/1, Comparator10/1, Comparator9/1, Comparator6/1, Comparator5/1, Comparator4/1, Comparator3/1, Comparator2/1, Comparator1/1, Comparator/1
  Comparator2/1 -> Add2/1
  Comparator11/1 -> Add6/2
  Add11/1 -> Add12/1
  Comparator1/1 -> Add1/2
  Constant22/1 -> Mux_inside_parenthesis 1/16
  Add3/1 -> Add10/2
  Add10/1 -> Add12/2
  Comparator12/1 -> Add7/1
  Comparator8/1 -> Add5/1
  Constant9/1 -> "Mux_Slope "/10
  Add7/1 -> Add8/2
  Add14/1 -> Delay1/1, Mux_inside_parenthesis 1/1
  Constant42/1 -> Mux_Slope 1/9
  Constant1/1 -> "Mux_Slope "/3
  Constant16/1 -> "Mux_Slope "/16
  Constant24/1 -> Mux_inside_parenthesis 1/4
  Constant19/1 -> Mux_inside_parenthesis 1/12
  Constant39/1 -> Mux_Slope 1/4
  Constant41/1 -> Mux_Slope 1/6
  Constant38/1 -> Mux_Slope 1/5
  Delay1/1 -> Delay2/1, "Mux_Slope "/1
  Constant30/1 -> Mux_inside_parenthesis 1/10
  Constant45/1 -> Mux_Slope 1/10
  Constant44/1 -> Mux_Slope 1/11
  Constant34/1 -> Mux_Slope 1/12
  Constant28/1 -> Mux_inside_parenthesis 1/8
  Constant26/1 -> Mux_inside_parenthesis 1/6
  Constant21/1 -> Mux_inside_parenthesis 1/14
  Constant8/1 -> "Mux_Slope "/11
  Constant12/1 -> "Mux_Slope "/12
  Constant10/1 -> "Mux_Slope "/13
  Comparator5/1 -> Add3/2
  Constant27/1 -> Mux_inside_parenthesis 1/9
  Constant18/1 -> Mux_inside_parenthesis 1/2
  Comparator4/1 -> Add3/1
  Comparator10/1 -> Add6/1
  Constant11/1 -> "Mux_Slope "/2
  "Mux_Slope "/1 -> Mult/2
  Constant15/1 -> Mux_inside_parenthesis 1/3
  Constant32/1 -> Mux_Slope 1/13
  Constant36/1 -> Mux_Slope 1/14
  Constant35/1 -> Mux_Slope 1/15
  Constant31/1 -> Mux_Slope 1/3
  Constant25/1 -> Mux_inside_parenthesis 1/7
  Constant37/1 -> Mux_Slope 1/16
  Constant33/1 -> Mux_Slope 1/2
  Constant43/1 -> Mux_Slope 1/8
  Constant40/1 -> Mux_Slope 1/7
  Delay2/1 -> Mux_Slope 1/1
  Mult/1 -> Add16/1
  Add1/1 -> Add11/2
  Add9/1 -> Add13/1
  Constant6/1 -> "Mux_Slope "/9
  Constant4/1 -> "Mux_Slope "/7
  Add5/1 -> Add9/2
  Comparator6/1 -> Add4/1
  Comparator7/1 -> Add4/2
  Comparator3/1 -> Add2/2
  Mux_Slope 1/1 -> Add16/2
  Add8/1 -> Add13/2
  Mux_inside_parenthesis 1/1 -> Add15/2
  Constant7/1 -> "Mux_Slope "/8
  Add15/1 -> Mult/1
  Delay3/1 -> Out1/1
  Add16/1 -> Delay3/1
